simulink model "testing_platform_continuous_reaction"  (Simulink 7.9)
settings: Solver=ode45  StartTime=0.0  StopTime=100  FixedStep=Ts  MaxStep=100  RelTol=1e-4
values from neighbouring files (symbols this model uses):
  coeff = block.DialogPrm(1).Data    [continuous_reaction_model.m]    (also in continuous_reaction_model_scaled.m; continuous_reaction_model_scaled_sensitivity.m)
  x0 = block.DialogPrm(2).Data    [continuous_reaction_model.m]    (also in continuous_reaction_model_scaled.m; continuous_reaction_model_scaled_sensitivity.m)
settings Model: Creator=mforgione  LastModifiedBy=marco  SimulationMode=accelerator
settings OptimizationCC: InitFltsAndDblsToZero=on  AccelVerboseBuild=on
settings DebuggingCC: FcnCallInpInsideContextMsg=Use local settings  StrictBusMsg=Warning
settings GRTTargetCC: CombineOutputUpdateFcns=off  GRTInterface=on

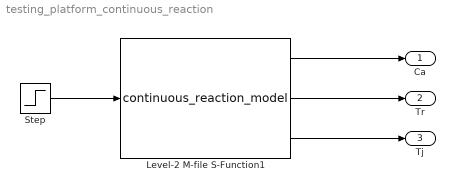
== system testing_platform_continuous_reaction ==
  Level-2 M-file S-Function1 : M-S-Function  FunctionName=continuous_reaction_model  Parameters=coeff x0
  Step : Step  Before=0.01  After=0.015  SampleTime=0
  Ca : Outport
  Tr : Outport  Port=2
  Tj : Outport  Port=3
  wires:
  Level-2 M-file S-Function1/1 -> Ca/1
  Level-2 M-file S-Function1/2 -> Tr/1
  Level-2 M-file S-Function1/3 -> Tj/1
  Step/1 -> Level-2 M-file S-Function1/1
